simulink model "HevIpsPowertrainController"  (R2025b)
settings: configuration reference "VehicleFixed10ms" (kept outside this file)
undefined symbols (not defined in the file): CtrlBcuTrlrBrkGain, CtrlVcuHevIpsBattChrgPwrMax, CtrlVcuHevIpsBattDischrgPwrMax, CtrlVcuHevIpsChrgLmtBpt, CtrlVcuHevIpsDischrgLmtBpt, CtrlVcuHevIpsEngPwr, CtrlVcuHevIpsEngSpd, CtrlVcuHevIpsEngTrq, CtrlVcuHevIpsEngTrqWhl, CtrlVcuHevIpsEVSpdLmt, CtrlVcuHevIpsGenPwrMax, CtrlVcuHevIpsGenTrqMax, CtrlVcuHevIpsMotPwr, CtrlVcuHevIpsN_idle, CtrlVcuHevIpsNsysWhl, CtrlVcuHevIpsRegenBrkCutOff, CtrlVcuHevIpsRegenBrkSpdBpt, CtrlVcuHevIpsSocBpt, CtrlVcuHevIpsSOCChrgFactor, CtrlVcuHevIpsSOCmin, CtrlVcuHevIpsSOCtarget, CtrlVcuHevIpsSysTrqWhl, PlntBrkActrBoreFrnt, PlntBrkFrntBias, PlntBrkKinFricCffFrnt, PlntBrkNumPadsFrnt, PlntBrkPadMeanRadiusFrnt, PlntBrkPrsFctr, PlntBrkRearBias, PlntDiffrntlRatio, PlntEM1EffTbl, PlntEM1Spd, PlntEM1SpdEff, PlntEM1Trq, PlntEM1TrqEff, PlntEM2EffTbl, PlntEM2Spd, PlntEM2SpdEff, PlntEM2Trq, PlntEM2TrqEff, PlntHevIpsP1SunRingRatio, PlntHevIpsP2GearRatio
libraries: simulink x19, autolibutils x4, slpidlib x1
(part 2 of 2)

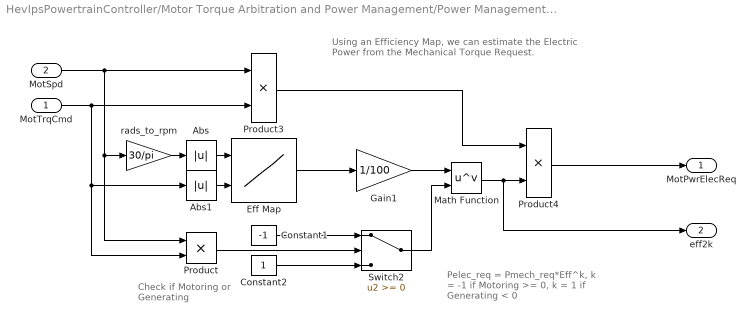
== system HevIpsPowertrainController/Motor Torque Arbitration and Power Management/Power Management/Mech to Elec Power Estimate ==
  note: Check if Motoring
      | or Generating
  note: Using an Efficiency Map, we can estimate the
      | Electric Power from the Mechanical  Torque Request.
  note: Pelec_req = Pmech_req*Eff^k,
      | k = -1 if Motoring >= 0,
      | k = 1 if Generating < 0
  MotTrqCmd : Inport
  MotSpd : Inport  Port=2
  Abs : Abs  SaturateOnIntegerOverflow=off
  Abs1 : Abs  SaturateOnIntegerOverflow=off
  Constant1 : Constant  Value=-1  SampleTime=-1
  Constant2 : Constant  SampleTime=-1
  Eff Map : Lookup_n-D  BreakpointsForDimension1=PlntEM1SpdEff*30/pi  BreakpointsForDimension2=PlntEM1TrqEff  Table=PlntEM1EffTbl  ExtrapMethod=Clip  UseLastTableValue=on  InternalRulePriority=Speed  OutDataTypeStr=Inherit: Inherit from 'Table data'  RndMeth=Simplest
      settings: InputPortMap=u0,u1
  Gain1 : Gain  Gain=1/100
  Math Function : Math  Operator=pow  SignedPower=on  OutputSignalType=real
  Product : Product
  Product3 : Product
  Product4 : Product
  Switch2 : Switch  SaturateOnIntegerOverflow=off  InputSameDT=off
  rads_to_rpm : Gain  Gain=30/pi
  MotPwrElecReq : Outport  VectorParamsAs1DForOutWhenUnconnected=off
  eff2k : Outport  Port=2  VectorParamsAs1DForOutWhenUnconnected=off
  wires:
  Product3/1 -> Product4/1
  Switch2/1 -> Math Function/2
  Constant1/1 -> Switch2/1
  Constant2/1 -> Switch2/3
  Eff Map/1 -> Gain1/1
  Abs/1 -> Eff Map/1
  Gain1/1 -> Math Function/1
  Math Function/1 -> eff2k/1, Product4/2
  Product4/1 -> MotPwrElecReq/1
  Abs1/1 -> Eff Map/2
  rads_to_rpm/1 -> Abs/1
  Product/1 -> Switch2/2
  MotSpd/1 -> Product3/1, Product/1, rads_to_rpm/1
  MotTrqCmd/1 -> Product3/2, Product/2, Abs1/1

== system HevIpsPowertrainController/Motor Torque Arbitration and Power Management/Power Management/Torque Limit ==
  MotTrq : Inport
  MotSpd : Inport  Port=2
  Gain : Gain  Gain=-1
  MaxMotTrqVsSpd : Lookup_n-D  NumberOfTableDimensions=1  BreakpointsForDimension1=PlntEM1Spd*30/pi  Table=PlntEM1Trq  ExtrapMethod=Clip  UseLastTableValue=on  InternalRulePriority=Speed  OutDataTypeStr=Inherit: Inherit from 'Table data'  RndMeth=Simplest
  Saturation Dynamic : simulink/Discontinuities/Saturation Dynamic  OutMin=[]  OutMax=[]  OutDataTypeStr=Inherit: Same as second input  OutDataType=fixdt(1, 16)  OutScaling=2^-10  DoSatur=off
  rads_to_rpm : Gain  Gain=30/pi
  MotTrqCmd : Outport  VectorParamsAs1DForOutWhenUnconnected=off
  wires:
  MotTrq/1 -> Saturation Dynamic/2
  Saturation Dynamic/1 -> MotTrqCmd/1
  MotSpd/1 -> rads_to_rpm/1
  MaxMotTrqVsSpd/1 -> Gain/1, Saturation Dynamic/1
  rads_to_rpm/1 -> MaxMotTrqVsSpd/1
  Gain/1 -> Saturation Dynamic/3

== stateflow chart HevIpsPowertrainController/IPS Supervisory Control ==
  settings: enableNonTerminalStates=1
  state Operating_Modes [parallel]
    entry, during:
    WhlPwrCmd = WhlTrqCmd*WhlSpd;
    SOCopt = (SOCtarget/100) - 0.5*VehMass*VehSpd*VehSpd*EffRechrg/BattEnergy;
    ChrgPwr = SOCChrgFactor*(SOCopt - SOC/100)*AccelPed;
    EngOnReq = EngOnCalc(SOC,BattPwr,BattPwrDischrgLmt,VehSpd,EVSpdLmt,AccelPed,WhlPwrCmd,SOCopt,OpMode);
    settings: executionOrder=1
    state Driving
      state HEV
        entry:
        InitFlag = 1;
        MotMode = 2;
        during:
        [Low,High] = ModeSelection(WhlSpd,WhlPwrCmd,AccelPed,ChrgPwr,BattPwrChrgLmt);
        exit:
        EngPwrCmd = 0;
        MotPwrCmd = 0;
        MotMode = 1;
        state Low_Power_Charge_Sustain
          entry:
          StateChange = 0;
          during:
          OpMode = 3;
          [EngPwrCmd,MotPwrCmd] = OpMode3(WhlPwrCmd,ChrgPwr,BattPwrChrgLmt,GenPwrCmd,EngTrqOut,EngSpd);
          state [EngPwrCmd,MotPwrCmd] = OpMode3(WhlPwrCmd,ChrgPwr,BattPwrChrgLmt,GenPwrCmd,EngTrqOut,EngSpd) [function]
        state High_Power_Charge_Deplete
          entry:
          InitFlag = 0;
          StateChange = 0;
          during:
          OpMode = 4;
          [EngPwrCmd,MotPwrCmd] = OpMode4(WhlTrqCmd,WhlSpd,WhlPwrCmd,EngTrqOut);
          state [EngPwrCmd,MotPwrCmd] = OpMode4(WhlTrqCmd,WhlSpd,WhlPwrCmd,EngTrqOut) [function]
        state Wait
          entry:
          StateChange = 1;
        state Wait1
          entry:
          StateChange = 1;
        state [Low,High] = ModeSelection(WhlSpd,WhlPwrCmd,AccelPed,ChrgPwr,BattPwrChrgLmt) [function]
        (default) -> Low_Power_Charge_Sustain
        Low_Power_Charge_Sustain -> High_Power_Charge_Deplete [order 1] : [High && InitFlag == 1 ]
        Operating_Modes.Driving.HEV.Wait -> High_Power_Charge_Deplete : [after(Ts,sec)]
        Low_Power_Charge_Sustain -> Operating_Modes.Driving.HEV.Wait [order 2] : [High && InitFlag == 0]
        Operating_Modes.Driving.HEV.Wait1 -> Low_Power_Charge_Sustain : [after(Ts,sec)]
        High_Power_Charge_Deplete -> Operating_Modes.Driving.HEV.Wait1 : [Low]
      state EV
        entry, during:
        OpMode = 1;
        EngPwrCmd = 0;
        MotMode = 1;
      state Wait
        entry, during:
        OpMode = 2;
        MotMode = 1;
      (default) -> EV
      EV -> Operating_Modes.Driving.Wait : [EngOnReq]
      Operating_Modes.Driving.Wait -> HEV [order 1] : [EngMode == 3]
      Operating_Modes.Driving.Wait -> EV [order 2] : [~EngOnReq]
      HEV -> EV : [~EngOnReq && EngMode == 1]
    state Wait1
      exit:
      StateChange = 1;
    state Stationary
      entry, during:
      Park = 1;
      exit:
      Park = 0;
      state No_Charge
        entry, during:
        OpMode = 5;
      state Charging
        entry, during:
        OpMode =6;
        EngPwrCmd = ChargePowerCalc(SOC);
        exit:
        EngPwrCmd = 0;
        state EngPwrCmd = ChargePowerCalc(SOC) [function]
      (default) -> No_Charge
      No_Charge -> Charging : [SOC < SOCmin]
      Charging -> No_Charge : [SOC >= SOCtarget]
    state EngOnReq = EngOnCalc(SOC,BattPwr,BattPwrDischrgLmt,VehSpd,EVSpdLmt,AccelPed,WhlPwrCmd,SOCopt,OpMode) [function]
    Stationary -> Driving : [AccelPed > 0.01]
    Driving -> Operating_Modes.Wait1 : [VehSpd < 0.05]
    Operating_Modes.Wait1 -> Driving [order 1] : [AccelPed > 0.1]
    Operating_Modes.Wait1 -> Stationary [order 2] : [after(2, sec)]
    (default) -> Stationary
  state Motor_Control [parallel]
    settings: executionOrder=2
    state Mot_EV
      entry, during:
      MotTrqCmd = MotTrqEV(WhlTrqCmd);
      state MotTrqCmd = MotTrqEV(WhlTrqCmd) [function]
    state Mot_HEV
      entry, during:
      MotTrqCmd = MotTrqHEV(MotPwrCmd,MotSpd);
      state MotTrqCmd = MotTrqHEV(MotPwrCmd,MotSpd) [function]
    (default) -> Mot_EV
    Mot_HEV -> Mot_EV : [MotMode == 1]
    Mot_EV -> Mot_HEV : [MotMode == 2]
  state Engine_Control [parallel]
    settings: executionOrder=4
    state Off
      entry, during:
      EngMode = 1;
      EngTrqCmd = 0;
      EngSpdCmd = 0;
      StateChange = 0;
    state Starting
      entry, during:
      StateChange = 0;
      EngMode = 2;
      EngTrqCmd = 0;
      EngSpdCmd = EngIdle;
      exit:
      StateChange = 1;
    state Run
      entry:
      StateChange = 1;
      during:
      StateChange = 0;
      EngMode = 3;
      [EngTrqCmd,EngSpdCmd] = TrqCalc(EngPwrCmd);
      state [EngTrqCmd,EngSpdCmd] = TrqCalc(EngPwrCmd) [function]
    state Wait
    (default) -> Off
    Off -> Starting : [EngOnReq]
    Starting -> Off [order 2] : [~EngOnReq]
    Engine_Control.Wait -> Off [order 2] : [after(1, sec)]
    Starting -> Run [order 1] : [abs(EngSpd - EngIdle) < 5 || EngSpd >= EngIdle]
    Run -> Engine_Control.Wait : [~EngOnReq]
    Engine_Control.Wait -> Run [order 1] : [EngOnReq]
  state Generator_Control [parallel]
    settings: executionOrder=3
    state OFF
      entry, during:
      % stay idle // do not start generator control
      EngSpdErr = 0;
      GenTrqCmd = 0;
      GenPwrCmd = 0;
    state wait
    state ON
      entry:
      StateChange = 0;
      during:
      % start and run generator control
      [EngSpdErr,GenTrqCmd,GenPwrCmd] = GenControl(GenSpd,EngSpd,BattPwrDischrgLmt,MotPwrElec,BattPwrChrgLmt,EngSpdCmd,EngMode);
      state [EngSpdErr,GenTrqCmd,GenPwrCmd] = GenControl(GenSpd,EngSpd,BattPwrDischrgLmt,MotPwrElec,BattPwrChrgLmt,EngSpdCmd,EngMode) [function]
    (default) -> OFF
    OFF -> wait : [VehSpd > 0.1 || GenSpd > 10]
    wait -> OFF [order 2] : [VehSpd < 0.05 && GenSpd < 10]
    ON -> OFF [order 1] : [VehSpd < 0.05 && GenSpd < 10]
    wait -> ON [order 1] : [after(Ts,sec)]
    ON -> wait [order 2] : [StateChange == 1]
  data: WhlPwrCmd function_input; ChrgPwr function_input; BattPwrChrgLmt function_input; EngPwrCmd function_output; GenPwrCmd function_input; MotPwrCmd function_output; EngTrqOut function_input; EngSpd function_input; WhlTrqCmd function_input; EngPwrCmd function_output; MotPwrCmd function_output; WhlSpd function_input; WhlPwrCmd function_input; EngTrqOut function_input; Low function_output; High function_output; WhlSpd function_input size=1; WhlPwrCmd function_input size=1; AccelPed function_input size=1; ChrgPwr function_input; BattPwrChrgLmt function_input; SOC function_input; EngPwrCmd function_output; SOC function_input; EngOnReq function_output; BattPwr function_input; BattPwrDischrgLmt function_input; VehSpd function_input; EVSpdLmt function_input; AccelPed function_input; WhlPwrCmd function_input; SOCopt function_input; OpMode function_input; WhlTrqCmd function_input; MotTrqCmd function_output; MotPwrCmd function_input; MotTrqCmd function_output; MotSpd function_input; EngPwrCmd function_input; EngTrqCmd function_output; EngSpdCmd function_output; GenSpd function_input; EngSpd function_input; EngSpdErr function_output; GenTrqCmd function_output; GenPwrCmd function_output; BattPwrDischrgLmt function_input; MotPwrElec function_input; BattPwrChrgLmt function_input; EngSpdCmd function_input; EngMode function_input; EVSpdLmt input; EngIdle input; SOCtarget input double =60; SOCmin input; SOCChrgFactor input double =150000; SOC input; OpMode output; MotMode output double; EngOnReq output; EngMode output double; EngSpdErr output double; EngPwrCmd output; MotPwrCmd output; EffRechrg constant double =0.6; BattEnergy constant double =4717440; VehMass constant double =1310; ChrgPwr output double; WhlPwrCmd output double; SOCopt output double; VehSpd input; MotSpd input; BattPwrDischrgLmt input; BattPwrChrgLmt input; AccelPed input; EngTrqOut input; GenSpd input; BattPwr input; EngSpd input; WhlTrqCmd input; WhlSpd input; EngSpdCmd output double; GenPwrCmd output double; Park output double; EngTrqCmd output double; GenTrqCmd output double; MotTrqCmd output double; MotPwrElec input; Low local double; High local double; Ts local double =10e-3; StateChange local double =0; InitFlag local double =0

== stateflow chart HevIpsPowertrainController/IPS Supervisory Control/Operating_Modes.EngOnCalc/Check Power/Timer ==
  state Wait
    du:
    Out = 0;
  state StartTimer
    du:
    Out = 0;
  state TimerDone
    du:
    Out = 1;
  (default) -> StartTimer
  StartTimer -> Wait : [In]
  Wait -> TimerDone [order 2] : after(0.1, sec)
  Wait -> StartTimer [order 1] : [In == 0]
  TimerDone -> StartTimer : [In == 0]
  data: In input; Out output
